simulink model "radar_subscription"  (R2020a)
settings: Solver=VariableStepAuto  StartTime=0.0  StopTime=inf  RelTol=1e-3
undefined symbols (not defined in the file): Acceleration, Steer
libraries: robotlib x3
settings Model: Creator=root  LastModifiedBy=root

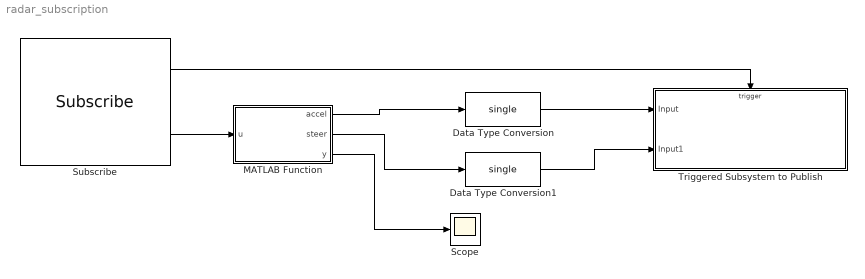
== system radar_subscription ==
  Data Type Conversion : DataTypeConversion  OutDataTypeStr=single
  Data Type Conversion1 : DataTypeConversion  OutDataTypeStr=single
  MATLAB Function : MATLAB Function  TreatAsAtomicUnit=on
  Scope : Scope
  Subscribe : robotlib/Subscribe  topicSource=Specify your own  topic=/radar_processed_array  messageType=radar_msgs/RadarProcessedArray  sampleTime=-1  messageQueueLength=1
  Triggered Subsystem to Publish : Subsystem  TreatAsAtomicUnit=on
  wires:
  Subscribe/2 -> MATLAB Function/1(u)
  MATLAB Function/1(accel) -> Data Type Conversion/1
  MATLAB Function/2(steer) -> Data Type Conversion1/1
  Subscribe/1 -> Triggered Subsystem to Publish/Trigger
  Data Type Conversion/1 -> Triggered Subsystem to Publish/1(Input)
  Data Type Conversion1/1 -> Triggered Subsystem to Publish/2(Input1)
  MATLAB Function/3(y) -> Scope/1

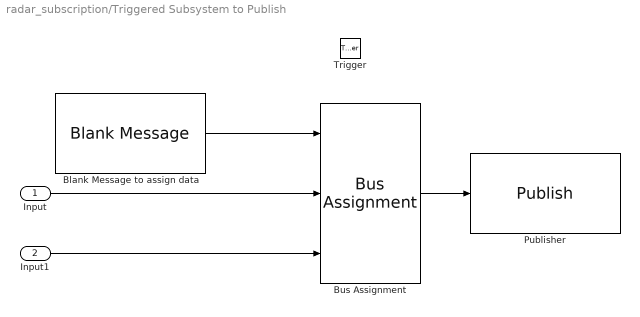
== system radar_subscription/Triggered Subsystem to Publish ==
  Input : Inport
  Input1 : Inport  Port=2
  Trigger : TriggerPort  VariantControl=Variant
  Blank Message to assign data : robotlib/Blank Message  messageClass=Message  entityType=ros_sut/ControlCommand  messageType=ros_sut/ControlCommand  SampleTime=inf
  Bus Assignment : BusAssignment  AssignedSignals=Acceleration,Steer
  Publisher : robotlib/Publish  topicSource=Select from ROS network  topic=/control_cmd  messageType=ros_sut/ControlCommand  messageQueueLength=1
  wires:
  Blank Message to assign data/1 -> Bus Assignment/1
  Bus Assignment/1 -> Publisher/1
  Input/1 -> Bus Assignment/2
  Input1/1 -> Bus Assignment/3

== matlab function radar_subscription/MATLAB Function ==
  data: u input; accel output; steer output; y output
function [accel, steer, y] = Range(u)
i = 1;
y = -10.0;


    while ( i < length(u.Groundtruth))
        range = u.Groundtruth(i,1).Range;
        object_type = u.Groundtruth(i,1).ObjectType;
        
        if (object_type == 2.0)
            y = range;
        end
        i = i + 1;
    end
    
    if y < 25
        accel = -100.0;
        steer = 0.0;
    else
        accel = 0.5;
        steer = 0.0;
    end
        
end
